simulink model "DC_DC_BuckBoostConverter"  (Simulink 7.0)
settings: Solver=ode23t  StartTime=0.0  StopTime=0.005  MaxStep=1.e-07  MinStep=1.e-10  RelTol=1e-3
libraries: powerlib x10, simulink x1
settings Model: Creator=sc  LastModifiedBy=sc
settings SolverCC: InitialStep=1.e-07

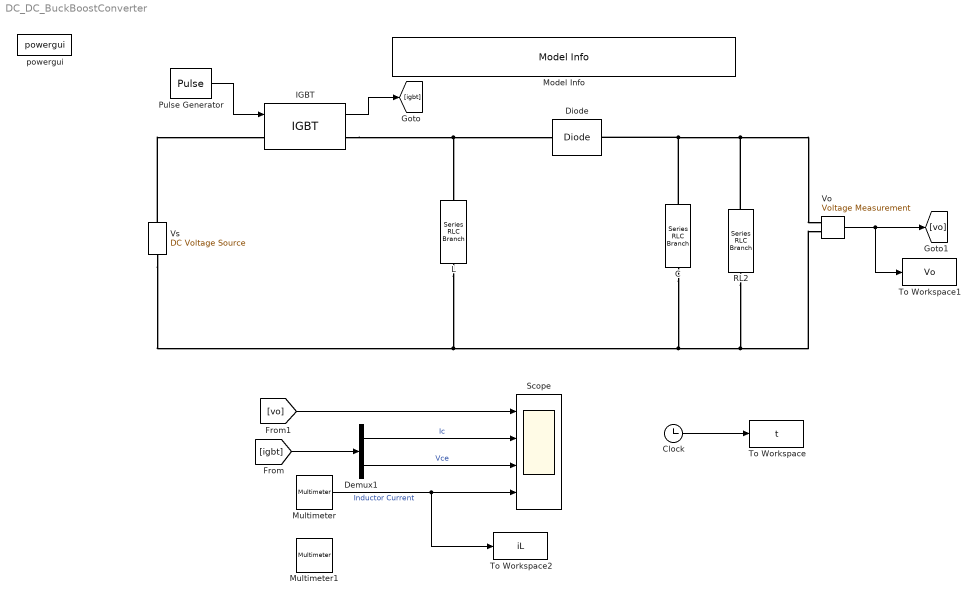
== system DC_DC_BuckBoostConverter ==
  " C" : powerlib/Elements/Series RLC Branch  Orientation=down  DialogController=POWERSYS.PowerSysDialog  PhysicalDomain=powersysdomain  SubClassName=unknown  LeftPortType=p1  RightPortType=p1  LConnTagsString=__new0  RConnTagsString=__new0  BranchType=C  Resistance=1.0  Inductance=1e-3  SetiL0=off  InitialCurrent=0  Capacitance=20.e-06  Setx0=off  InitialVoltage=0  Measurements=Branch current
  " L" : powerlib/Elements/Series RLC Branch  Orientation=down  DialogController=POWERSYS.PowerSysDialog  PhysicalDomain=powersysdomain  SubClassName=unknown  LeftPortType=p1  RightPortType=p1  LConnTagsString=__new0  RConnTagsString=__new0  BranchType=L  Resistance=1.0  Inductance=200.e-6  SetiL0=off  InitialCurrent=0  Capacitance=1.0  Setx0=off  InitialVoltage=0  Measurements=Branch current
  " RL2" : powerlib/Elements/Series RLC Branch  Orientation=down  DialogController=POWERSYS.PowerSysDialog  PhysicalDomain=powersysdomain  SubClassName=unknown  LeftPortType=p1  RightPortType=p1  LConnTagsString=__new0  RConnTagsString=__new0  BranchType=R  Resistance=10  Inductance=1e-3  SetiL0=off  InitialCurrent=0  Capacitance=1.e-04  Setx0=off  InitialVoltage=0  Measurements=Branch voltage
  Clock : Clock
      settings: Decimation=10
  Demux1 : Demux  Outputs=2
  Diode : powerlib/Power Electronics/Diode  Orientation=left  DialogController=POWERSYS.PowerSysDialog  SystemSampleTime=-1  Ron=0.01  Lon=0  Vf=0.8  IC=0  Rs=1000  Cs=inf  Measurements=off
  IGBT : powerlib/Power Electronics/IGBT  DialogController=POWERSYS.PowerSysDialog  SystemSampleTime=-1  Ron=0.001  Lon=0  Vf=1  Tf=1e-7  Tt=1e-7  IC=0  Rs=100  Cs=1.e-07  Measurements=on
  Model Info : simulink/Model-Wide Utilities/Model Info  SystemSampleTime=-1  InitialBlockCM=None  BlockCM=None  Frame=on  DisplayStringWithTags=DC-DC BuckBoost Converter  HorizontalTextAlignment=Center  LeftAlignmentValue=0.5  SourceBlockDiagram=DC_DC_BuckBoostConverter  TagMaxNumber=20
  Multimeter : powerlib/Measurements/Multimeter  SystemSampleTime=-1  PhasorSimulation=off  OutputType=Complex  sel=2  L=3  Gain=1  yselected="{'Ib:  L'};"  PSBOutputType=1  PSBequivalent=0  AxesSetting=[0,0.1,-100,100]  Display=0  SavedBlockNames=-11
  Multimeter1 : powerlib/Measurements/Multimeter  SystemSampleTime=-1  PhasorSimulation=off  OutputType=Complex  sel=[1 3 2]  L=3  Gain=[1 -1 1]  yselected="{'Ub:  RL2','Ib:  C','Ib:  L'};"  PSBOutputType=1  PSBequivalent=0  AxesSetting=[0,0.1,-100,100]  Display=1  SavedBlockNames=-11
  Pulse Generator : DiscretePulseGenerator  PulseType=Time based  Period=5.e-05  PulseWidth=60
  Scope : Scope  NumInputPorts=4
      settings: TimeRange=0.005  YMin=-50~-50~-50~0  YMax=150~100~150~60  SaveName=var  MaxDataPoints=100000
  To Workspace : ToWorkspace  VariableName=t  SampleTime=-1  SaveFormat=Array
  To Workspace1 : ToWorkspace  VariableName=Vo  SampleTime=-1  SaveFormat=Array
  To Workspace2 : ToWorkspace  VariableName=iL  SampleTime=-1  SaveFormat=Array
  Vo : powerlib/Measurements/Voltage Measurement  DialogController=POWERSYS.PowerSysDialog  SystemSampleTime=-1  PhasorSimulation=off  OutputType=Complex  PSBequivalent=0
  Vs : powerlib/Electrical Sources/DC Voltage Source  Orientation=up  DialogController=POWERSYS.PowerSysDialog  SystemSampleTime=-1  Amplitude=100  Measurements=None
  powergui : powerlib/powergui  SystemSampleTime=-1  SimulationMode=Continuous  SampleTime=50e-6  echomessages=off  RestoreLinks=warning  x0status=blocks  Frange=[0:2:500]  Ylog=off  Xlog=on  ShowGrid=off  save=off  variable=ZData  ZoomFFT=on  StartTime=0.0  cycles=1  DisplayStyle=1  fundamental=60  FreqAxis=off  MaxFrequency=1000  frequencyindice=0  frequencyindicesteady=1  RmsSteady=1  display=off  Ts=0  frequency=60  methode=off  HookPort=off  Interpol=off  SPID=off  FunctionMessages=off
  wires:
  [igbt] -> Demux1/1
  Vo/1 -> [vo], To Workspace1/1
  [vo] -> Scope/1
  Demux1/1 -> Scope/2  "Ic"
  Demux1/2 -> Scope/3  "Vce"
  Multimeter/1 -> Scope/4, To Workspace2/1  "Inductor Current"
  Clock/1 -> To Workspace/1
  IGBT/1 -> [igbt]
  Pulse Generator/1 -> IGBT/1
  connections:
  Vs/LConn1 -- Vo/LConn2 -- " RL2"/RConn1 -- " C"/RConn1 -- " L"/RConn1
  " C"/LConn1 -- " RL2"/LConn1 -- Vo/LConn1 -- Diode/LConn1
  Vs/RConn1 -- IGBT/LConn1
  IGBT/RConn1 -- Diode/RConn1 -- " L"/LConn1
